simulink model "araba_pozisyon_on_off_kontrol"  (Simulink 10.1)
settings: Solver=FixedStepAuto  StartTime=0.0  StopTime=stopTime  FixedStep=T  RelTol=1e-3
values from neighbouring files (symbols this model uses):
  A = 10000    [init_RC_devresi_bang_bang_kontrol.m]    (also in init_araba_hiz_kontrol.m = [0 1; 0 -b/m]; init_araba_hiz_on_off_kontrol.m = [0 1; 0 -b/m]; init_araba_hiz_pid_kontrol.m = [0 1; 0 -b/m]; init_araba_pozisyon_bang_bang_kontrol.m = [0 1; 0 -b/m])
  b = 50    [init_araba_hiz_kontrol.m]    (also in init_araba_hiz_on_off_kontrol.m; init_araba_hiz_pid_kontrol.m; init_araba_pozisyon_bang_bang_kontrol.m = 250; init_araba_pozisyon_kontrol.m)
  B = [0; 1/m]    [init_araba_hiz_kontrol.m]    (also in init_araba_hiz_on_off_kontrol.m; init_araba_hiz_pid_kontrol.m; init_araba_pozisyon_bang_bang_kontrol.m; init_araba_pozisyon_kontrol.m)
  C = 1e-4    (= 0.0001)    [init_RC_devresi.m]    (also in init_RC_devresi_bang_bang_kontrol.m; init_araba_hiz_kontrol.m = [0 1]; init_araba_hiz_on_off_kontrol.m = [0 1]; init_araba_hiz_pid_kontrol.m = [0 1])
  D = 0    [init_araba_hiz_kontrol.m]    (also in init_araba_hiz_on_off_kontrol.m; init_araba_hiz_pid_kontrol.m; init_araba_pozisyon_bang_bang_kontrol.m; init_araba_pozisyon_kontrol.m)
  K = 10000    [init_araba_hiz_on_off_kontrol.m]    (also in init_araba_pozisyon_bang_bang_kontrol.m = 70000; init_araba_pozisyon_on_off_kontrol.m = 5000)
  m = 1000    [init_araba_hiz_kontrol.m]    (also in init_araba_hiz_on_off_kontrol.m; init_araba_hiz_pid_kontrol.m; init_araba_pozisyon_bang_bang_kontrol.m; init_araba_pozisyon_kontrol.m)
  r = 5    [init_RC_devresi_bang_bang_kontrol.m]    (also in init_araba_hiz_kontrol.m = 90; init_araba_hiz_on_off_kontrol.m = 90; init_araba_hiz_pid_kontrol.m = 90; init_araba_pozisyon_bang_bang_kontrol.m = 1000)
  x10 = 0    [init_araba_hiz_kontrol.m]    (also in init_araba_hiz_on_off_kontrol.m; init_araba_hiz_pid_kontrol.m; init_araba_pozisyon_bang_bang_kontrol.m; init_araba_pozisyon_kontrol.m)
  x20 = 0    [init_araba_hiz_kontrol.m]    (also in init_araba_hiz_on_off_kontrol.m; init_araba_hiz_pid_kontrol.m; init_araba_pozisyon_bang_bang_kontrol.m; init_araba_pozisyon_kontrol.m)
undefined symbols (not defined in the file or in its folder): sgn
settings Model: Creator=TULPAR  LastModifiedBy=TULPAR
settings DataIOCC: SaveFormat=Dataset  ReturnWorkspaceOutputs=on
settings OptimizationCC: LifeSpan=auto
settings DebuggingCC: UnderspecifiedInitializationDetection=Simplified  MergeDetectMultiDrivingBlocksExec=error  SFUnexpectedBacktrackingDiag=error  SFNoUnconditionalDefaultTransitionDiag=error  SFExecutionAtInitializationDiag=warning  ArithmeticOperatorsInVariantConditions=error
settings HardwareCC: ProdBitPerPointer=64  ProdBitPerSizeT=64  ProdBitPerPtrDiffT=64  ProdLargestAtomicFloat=Float  ProdIntDivRoundTo=Zero  ProdEndianess=LittleEndian  ProdWordSize=64  ProdHWDeviceType=Intel->x86-64 (Windows64)
settings ModelReferenceCC: PropagateSignalLabelsOutOfModel=on
settings SFSimCC: SimUseLocalCustomCode=on  CustomCodeUndefinedFunction=FilterOut
settings RTWCC: RTWUseLocalCustomCode=on
settings CodeAppCC: StateflowObjectComments=off
settings GRTTargetCC: TargetLangStandard=C99 (ISO)  CombineOutputUpdateFcns=on  GRTInterface=off
settings ConfigComp: CovMetricSettings=dwe  CovHtmlReporting=off  CovSaveCumulativeToWorkspaceVar=off  CovSaveSingleToWorkspaceVar=off  CovExternalEMLEnable=on

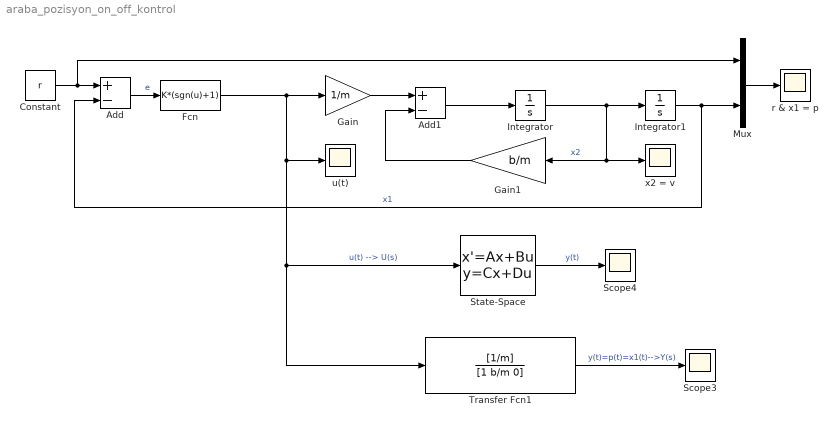
== system araba_pozisyon_on_off_kontrol ==
  Add : Sum  Inputs=+-
  Add1 : Sum  Inputs=+-
  Constant : Constant  Value=r
  Fcn : Fcn  Expr=K*(sgn(u)+1)
  Gain : Gain  Gain=1/m
  Gain1 : Gain  Gain=b/m
  Integrator : Integrator  InitialCondition=x20
  Integrator1 : Integrator  InitialCondition=x10
  Mux : Mux  Inputs=2
  Scope3 : Scope
  Scope4 : Scope
  State-Space : StateSpace  A=A  B=B  C=C  D=D  InitialCondition=[x10 x20]
  Transfer Fcn1 : TransferFcn  Numerator=[1/m]  Denominator=[1 b/m 0]
  r & x1 = p : Scope
  u(t) : Scope
  x2 = v : Scope
  wires:
  Fcn/1 -> u(t)/1, State-Space/1, Transfer Fcn1/1, Gain/1  "u(t) --> U(s)"
  State-Space/1 -> Scope4/1  "y(t)"
  Integrator1/1 -> Mux/2, Add/2  "x1"
  Transfer Fcn1/1 -> Scope3/1  "y(t)=p(t)=x1(t)-->Y(s)"
  Integrator/1 -> Gain1/1, x2 = v/1, Integrator1/1  "x2"
  Add1/1 -> Integrator/1
  Gain/1 -> Add1/1
  Constant/1 -> Mux/1, Add/1
  Add/1 -> Fcn/1  "e"
  Gain1/1 -> Add1/2
  Mux/1 -> r & x1 = p/1
